simulink library "SUS_IOP_WD_2_DC_RMS"  (Simulink 8.0)
settings: Solver=ode45  StartTime=0.0  StopTime=10.0  RelTol=1e-3
libraries: OSEM_WD_2_OUTPUTS x6
settings Model: Creator=controls  LastModifiedBy=controls

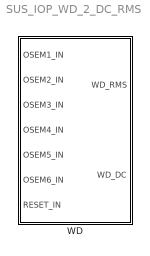
== system SUS_IOP_WD_2_DC_RMS ==
  WD : Subsystem

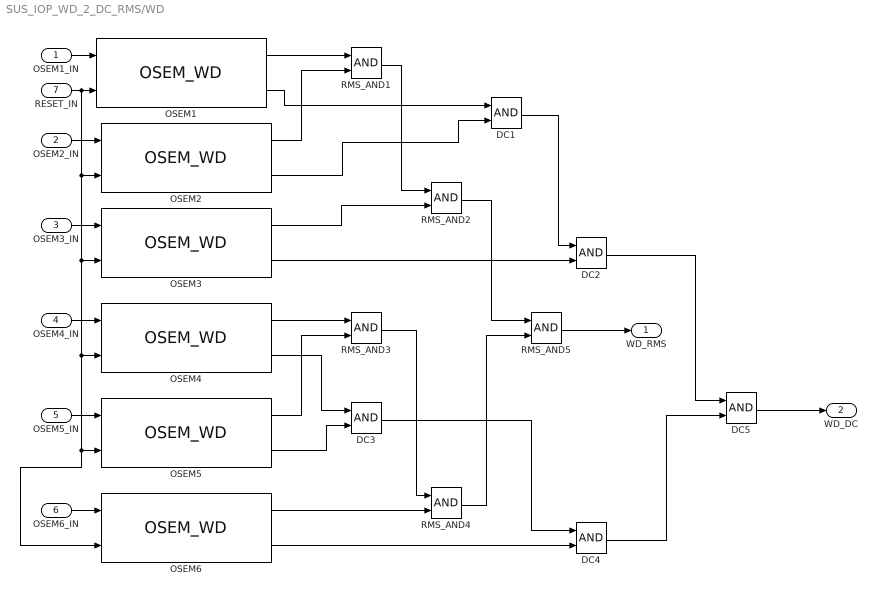
== system SUS_IOP_WD_2_DC_RMS/WD ==
  OSEM1_IN : Inport
  OSEM2_IN : Inport  Port=2
  OSEM3_IN : Inport  Port=3
  OSEM4_IN : Inport  Port=4
  OSEM5_IN : Inport  Port=5
  OSEM6_IN : Inport  Port=6
  RESET_IN : Inport  Port=7
  DC{1..5} (5 alike) : Logic  AllPortsSameDT=off  OutDataTypeStr=boolean
  OSEM{1..6} (6 alike) : OSEM_WD_2_OUTPUTS/OSEM_WD
  RMS_AND{1..5} (5 alike) : Logic  AllPortsSameDT=off  OutDataTypeStr=boolean
  WD_RMS : Outport
  WD_DC : Outport  Port=2
  wires:
  OSEM1_IN/1 -> OSEM1/1
  OSEM2_IN/1 -> OSEM2/1
  OSEM3_IN/1 -> OSEM3/1
  OSEM4_IN/1 -> OSEM4/1
  OSEM5_IN/1 -> OSEM5/1
  OSEM6_IN/1 -> OSEM6/1
  RMS_AND1/1 -> RMS_AND2/1
  RMS_AND2/1 -> RMS_AND5/1
  RMS_AND5/1 -> WD_RMS/1
  RESET_IN/1 -> OSEM1/2, OSEM2/2, OSEM3/2, OSEM4/2, OSEM6/2, OSEM5/2
  OSEM1/1 -> RMS_AND1/1
  OSEM2/1 -> RMS_AND1/2
  OSEM3/1 -> RMS_AND2/2
  RMS_AND3/1 -> RMS_AND4/1
  OSEM4/1 -> RMS_AND3/1
  OSEM5/1 -> RMS_AND3/2
  OSEM6/1 -> RMS_AND4/2
  RMS_AND4/1 -> RMS_AND5/2
  OSEM1/2 -> DC1/1
  OSEM2/2 -> DC1/2
  OSEM3/2 -> DC2/2
  DC1/1 -> DC2/1
  OSEM4/2 -> DC3/1
  OSEM5/2 -> DC3/2
  OSEM6/2 -> DC4/2
  DC3/1 -> DC4/1
  DC4/1 -> DC5/2
  DC2/1 -> DC5/1
  DC5/1 -> WD_DC/1
